simulink model "problema_lqr"  (R2023b)
settings: Solver=VariableStepAuto  StartTime=0.0  StopTime=60  MaxStep=1e-3  RelTol=1e-3
values from neighbouring files (symbols this model uses):
  A = [-0.313, 56.7 0; -0.0139 -0.426 0; 0 56.7 0]    [CO_laborator_03.m]
  B = [0.232; 0.0203; 0]    [CO_laborator_03.m]
  K = lqr(A,B,Q,R)    [CO_laborator_03.m]
settings Model: Creator=ovidiuceoca  LastModifiedBy=ovidiuceoca

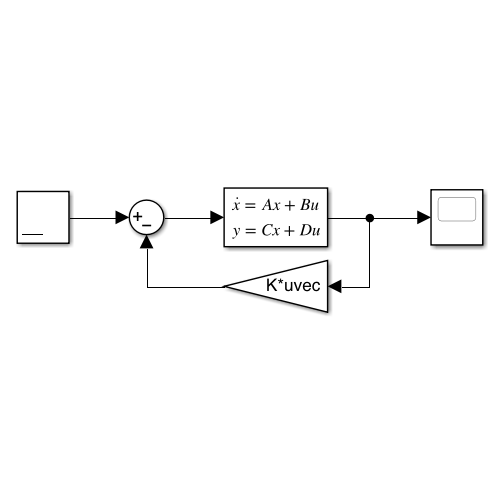
[thumbnail: Simulink's stored preview of the top-level diagram]
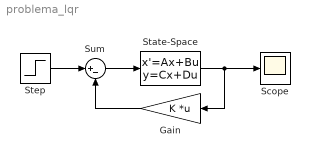
== system problema_lqr ==
  Gain : Gain  Gain=K  Multiplication=Matrix(K*u) (u vector)
  Scope : Scope
  State-Space : StateSpace  A=A  B=B  C=eye(3)  D=[0;0;0]  InitialCondition=[1;2;3]
  Step : Step  SampleTime=0
  Sum : Sum  Inputs=|+-
  wires:
  Gain/1 -> Sum/2
  State-Space/1 -> Scope/1, Gain/1
  Sum/1 -> State-Space/1
  Step/1 -> Sum/1
